simulink model "Sens_UltraStick25e"  (R2016b)
settings: Solver=VariableStepAuto  StartTime=0.0  StopTime=10.0  RelTol=1e-3
libraries: SensLib x3
settings Model: Creator=UAVLAB  LastModifiedBy=rega0051
settings DataIOCC: SaveOutput=off  SignalLogging=off  DSMLogging=off  SaveTime=off

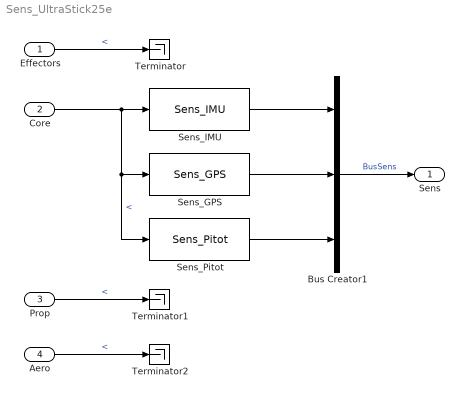
== system Sens_UltraStick25e ==
  Effectors : Inport  OutDataTypeStr=Bus: BusEff
      settings: AttributesFormatString=%<OutDataTypeStr>
  Core : Inport  Port=2  OutDataTypeStr=Bus: BusCore
      settings: AttributesFormatString=%<OutDataTypeStr>
  Prop : Inport  Port=3  OutDataTypeStr=Bus: BusProp
      settings: AttributesFormatString=%<OutDataTypeStr>
  Aero : Inport  Port=4  OutDataTypeStr=Bus: BusAero
      settings: AttributesFormatString=%<OutDataTypeStr>
  Bus Creator1 : BusCreator  Inputs=3  OutDataTypeStr=Bus: BusSens
      settings: AttributesFormatString=%<OutDataTypeStr>  InheritFromInputs=off
  Sens_GPS : SensLib/Sens_GPS  VariantControl=Variant1  sens=AC.GPS
  Sens_IMU : SensLib/Sens_IMU  VariantControl=VarImu_LocTransErr  sens=AC.IMU
  Sens_Pitot : SensLib/Sens_Pitot  VariantControl=VarAirData_LocTransErr  sens=AC.Pitot
  Terminator : Terminator
  Terminator1 : Terminator
  Terminator2 : Terminator
  Sens : Outport  OutDataTypeStr=Bus: BusSens
      settings: AttributesFormatString=%<OutDataTypeStr>
  wires:
  Core/1 -> Sens_Pitot/1, Sens_GPS/1, Sens_IMU/1  "<"
  Bus Creator1/1 -> Sens/1  "BusSens"
  Sens_GPS/1 -> Bus Creator1/2
  Sens_Pitot/1 -> Bus Creator1/3
  Sens_IMU/1 -> Bus Creator1/1
  Effectors/1 -> Terminator/1  "<"
  Prop/1 -> Terminator1/1  "<"
  Aero/1 -> Terminator2/1  "<"
